simulink model "single_PID_Inverted_pendulum_Swingup"  (R2023b)
settings: Solver=FixedStepDiscrete  StartTime=0.0  StopTime=inf  FixedStep=0.005  RelTol=1e-3
undefined symbols (not defined in the file): Kd0, Ki0, Kp0
libraries: simulink x9, arduinolib x2, slpidlib x1
settings Model: ExtModeTrigDuration=2  Creator=ADMIN  LastModifiedBy=giabaomai
settings SolverCC: AutoInsertRateTranBlk=on
settings OptimizationCC: EnhancedBackFolding=on  PassReuseOutputArgsAs=Individual arguments  ZeroExternalMemoryAtStartup=off  ZeroInternalMemoryAtStartup=off  MaxStackSize=64  OptimizeBlockOrder=speed  DifferentSizesBufferReuse=on  EfficientTunableParamExpr=on
settings DebuggingCC: MultiTaskCondExecSysMsg=none  ParameterPrecisionLossMsg=none  ParameterTunabilityLossMsg=error
settings HardwareCC: ProdBitPerInt=16  ProdBitPerPointer=16  ProdBitPerSizeT=16  ProdBitPerPtrDiffT=16  ProdLargestAtomicFloat=None  ProdWordSize=8  ProdHWDeviceType=Atmel->AVR
settings SFSimCC: MATLABDynamicMemAlloc=off
settings RTWCC: Description=Embedded Coder  SystemTargetFile=ert.tlc  HardwareBoard=Arduino Mega 2560  TemplateMakefile=ert_default_tmf  Toolchain=Arduino AVR  BuildConfiguration=Faster Runs
settings CodeAppCC: ForceParamTrailComments=on  IgnoreCustomStorageClasses=off  OperatorAnnotations=on  SimulinkDataObjDesc=on  SFDataObjDesc=on  InsertBlockDesc=on
settings ERTTargetCC: SupportContinuousTime=on  SupportVariableSizeSignals=on  ExtModeTransport=3  ExtModeStaticAlloc=on  ExtModeAutomaticAllocSize=off  ExtModeStaticAllocSize=2048  ExtModeMexFile=ext_xcp  ExtModeIntrfLevel=Level2 - Open

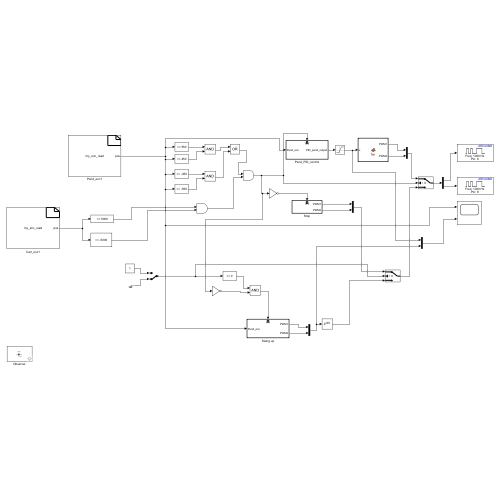
[thumbnail: Simulink's stored preview of the top-level diagram]
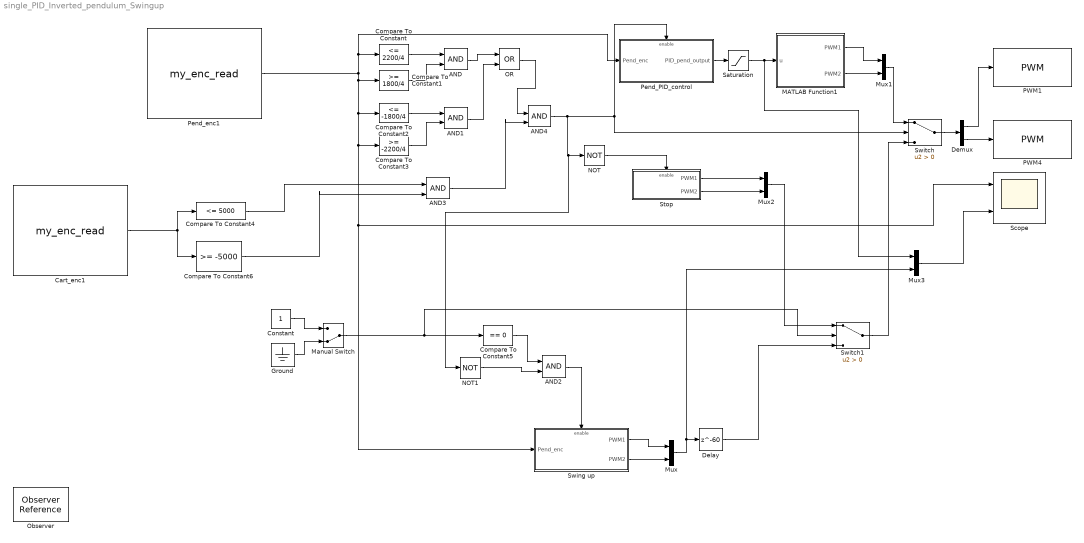
== system single_PID_Inverted_pendulum_Swingup ==
  AND : Logic  AllPortsSameDT=off  OutDataTypeStr=boolean
  AND1 : Logic  AllPortsSameDT=off  OutDataTypeStr=boolean
  AND2 : Logic  AllPortsSameDT=off  OutDataTypeStr=boolean
  AND3 : Logic  IconShape=distinctive  AllPortsSameDT=off  OutDataTypeStr=boolean
  AND4 : Logic  IconShape=distinctive  AllPortsSameDT=off  OutDataTypeStr=boolean
  Cart_enc1 : S-Function  FunctionName=my_enc_read  Parameters=uint8(3),uint8(2),uint8(0)  SFunctionModules=my_enc_read_wrapper.c  SFunctionDeploymentMode=off  EnableBusSupport=off  mask(S-Function Builder){}
      mask help: Simulink:masks:SFunctionBuilder_MD
      mask init:
      | val = [[.9  0.75 0.75 1 1 .9 .9 1]',[1 1 0.75 0.75 .9 .9 1 .9]'];try , sys = get_param(gcb,'SfunBuilderFcnName');if isempty(sys), sys = get_param(gcb,'FunctionName'); end,catch, sys = get_param(gcb,'FunctionName'); end
      settings: CopyFcn=set_param(gcbh,'LinkStatus','none')  OpenFcn=sfunctionwizard(gcbh)
      mask Display: plot(val(:,1),val(:,2)),disp(sys),port_label('output',1,'pos')
  Compare To Constant : simulink/Logic and Bit Operations/Compare To Constant  relop=<=  const=2200/4  OutDataTypeStr=boolean
  Compare To Constant1 : simulink/Logic and Bit Operations/Compare To Constant  relop=>=  const=1800/4  OutDataTypeStr=boolean
  Compare To Constant2 : simulink/Logic and Bit Operations/Compare To Constant  relop=<=  const=-1800/4  OutDataTypeStr=boolean
  Compare To Constant3 : simulink/Logic and Bit Operations/Compare To Constant  relop=>=  const=-2200/4  OutDataTypeStr=boolean
  Compare To Constant4 : simulink/Logic and Bit Operations/Compare To Constant  relop=<=  const=5000  OutDataTypeStr=boolean
  Compare To Constant5 : simulink/Logic and Bit Operations/Compare To Constant  relop===  const=0  OutDataTypeStr=boolean
  Compare To Constant6 : simulink/Logic and Bit Operations/Compare To Constant  relop=>=  const=-5000  OutDataTypeStr=boolean
  Constant : Constant
  Delay : Delay  DelayLength=60  SampleTime=0.005
  Demux : Demux  Outputs=2
  Ground : Ground
  MATLAB Function1 : MATLAB Function  TreatAsAtomicUnit=on
  Manual Switch : ManualSwitch  CurrentSetting=0
  Mux{,1..3} (4 alike) : Mux  Inputs=2
  NOT : Logic  Operator=NOT  IconShape=distinctive  AllPortsSameDT=off  OutDataTypeStr=boolean
  NOT1 : Logic  Operator=NOT  IconShape=distinctive  AllPortsSameDT=off  OutDataTypeStr=boolean
  OR : Logic  Operator=OR  AllPortsSameDT=off  OutDataTypeStr=boolean
  Observer : ObserverReference  ObserverModelName=single_PID_Inverted_pendulum_Swingup_Observer1
  PWM1 : arduinolib/PWM  pinNumber=6  frequencyType=Specify  desiredFrequency=1000  achievableFrequency=1000
  PWM4 : arduinolib/PWM  pinNumber=8  frequencyType=Specify  desiredFrequency=1000  achievableFrequency=1000
  Pend_PID_control : Subsystem  TreatAsAtomicUnit=on
  Pend_enc1 : S-Function  FunctionName=my_enc_read  Parameters=uint8(18),uint8(19),uint8(1)  SFunctionModules=my_enc_read_wrapper.c  SFunctionDeploymentMode=off  EnableBusSupport=off  mask(S-Function Builder){}
      mask help: Simulink:masks:SFunctionBuilder_MD
      mask init: same as single_PID_Inverted_pendulum_Swingup/Cart_enc1
      settings: CopyFcn=set_param(gcbh,'LinkStatus','none')  OpenFcn=sfunctionwizard(gcbh)
      mask Display:
      | plot(val(:,1),val(:,2))
      | disp(sys)
      | port_label('output',1,'pos')
  Saturation : Saturate  UpperLimit=255  LowerLimit=-255
  Scope : Scope  NumInputPorts=2
  Stop : Subsystem  TreatAsAtomicUnit=on
  Swing up : Subsystem  TreatAsAtomicUnit=on
  Switch : Switch  Criteria=u2 > Threshold  SaturateOnIntegerOverflow=off  InputSameDT=off
  Switch1 : Switch  Criteria=u2 > Threshold  SaturateOnIntegerOverflow=off  InputSameDT=off
  wires:
  MATLAB Function1/1(PWM1) -> Mux1/1
  Saturation/1 -> Mux3/1, MATLAB Function1/1(u)
  MATLAB Function1/2(PWM2) -> Mux1/2
  Pend_PID_control/1(PID_pend_output) -> Saturation/1
  Pend_enc1/1 -> Pend_PID_control/1(Pend_enc), Compare To Constant/1, Swing up/1(Pend_enc), Scope/1, Compare To Constant3/1, Compare To Constant2/1, Compare To Constant1/1
  Compare To Constant/1 -> AND/1
  Compare To Constant1/1 -> AND/2
  Compare To Constant2/1 -> AND1/1
  Compare To Constant3/1 -> AND1/2
  AND/1 -> OR/1
  AND1/1 -> OR/2
  NOT/1 -> Stop/Enable
  Stop/1(PWM1) -> Mux2/1
  Stop/2(PWM2) -> Mux2/2
  Mux1/1 -> Switch/1
  Switch/1 -> Demux/1
  Demux/1 -> PWM1/1
  Demux/2 -> PWM4/1
  Compare To Constant5/1 -> AND2/1
  NOT1/1 -> AND2/2
  Manual Switch/1 -> Switch1/2, Compare To Constant5/1
  AND2/1 -> Swing up/Enable
  Ground/1 -> Manual Switch/2
  Constant/1 -> Manual Switch/1
  Mux/1 -> Mux3/2, Delay/1
  Swing up/1(PWM1) -> Mux/1
  Swing up/2(PWM2) -> Mux/2
  Delay/1 -> Switch1/3
  Mux2/1 -> Switch1/1
  Switch1/1 -> Switch/3
  Mux3/1 -> Scope/2
  Cart_enc1/1 -> Compare To Constant4/1, Compare To Constant6/1
  Compare To Constant4/1 -> AND3/1
  Compare To Constant6/1 -> AND3/2
  OR/1 -> AND4/1
  AND3/1 -> AND4/2
  AND4/1 -> NOT1/1, NOT/1, Pend_PID_control/Enable, Switch/2

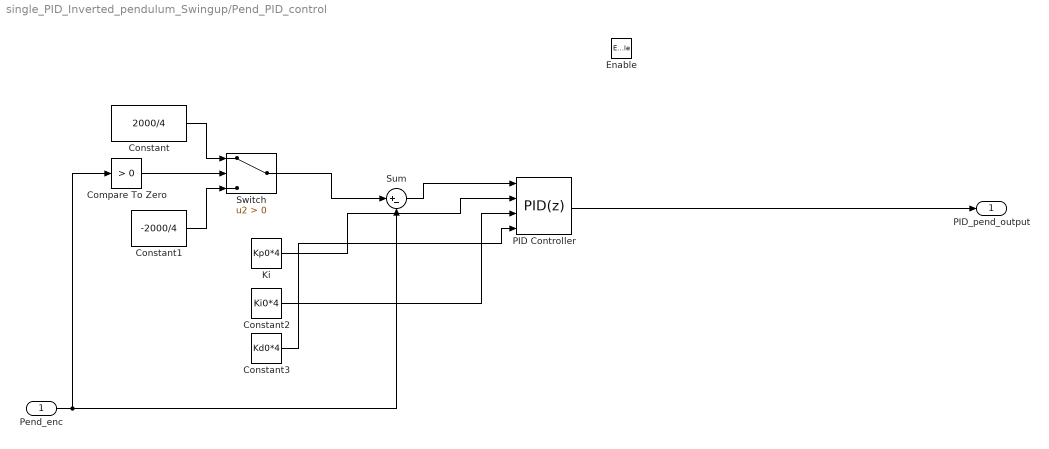
== system single_PID_Inverted_pendulum_Swingup/Pend_PID_control ==
  Pend_enc : Inport
  Enable : EnablePort
  Compare To Zero : simulink/Logic and Bit Operations/Compare To Zero  relop=>  OutDataTypeStr=boolean
  Constant : Constant  Value=2000/4
  Constant1 : Constant  Value=-2000/4
  Constant2 : Constant  Value=Ki0*4
  Constant3 : Constant  Value=Kd0*4
  Ki : Constant  Value=Kp0*4
  PID Controller : slpidlib/PID Controller  Controller=PID  Form=Parallel  TimeDomain=Discrete-time  UseExternalTs=off  SampleTime=0.005  IntegratorMethod=Backward Euler  FilterMethod=Forward Euler  ControllerParametersSource=external  P=0.35  I=0.12  UseKiTs=off  D=0.1  N=100  UseFilter=off  TunerSelectOption=Transfer Function Based (PID Tuner App)  ZeroCross=off  InitialConditionSource=internal  InitialConditionForIntegrator=0  InitialConditionForFilter=0  DifferentiatorICPrevScaledInput=0  ExternalReset=none  TrackingMode=off  Kt=1  LimitOutput=off  SatLimitsSource=internal  UpperSaturationLimit=255  LowerSaturationLimit=-255  LinearizeAsGain=off  AntiWindupMode=back-calculation  Kb=0.1  LimitIntegrator=off  UpperIntegratorSaturationLimit=inf  LowerIntegratorSaturationLimit=-inf  PGainOutDataTypeStr=Inherit: Match scaling  PProdOutDataTypeStr=Inherit: Match scaling  POutMin=[]  POutMax=[]  IOutMin=[]  IOutMax=[]  DOutMin=[]  DOutMax=[]  NOutMin=[]  NOutMax=[]  SumOutMin=[]  SumOutMax=[]  SaturationOutMin=[]  SaturationOutMax=[]  PParamMin=[]  PParamMax=[]  IParamMin=[]  IParamMax=[]  DParamMin=[]  DParamMax=[]  NParamMin=[]  NParamMax=[]  KbParamMin=[]  KbParamMax=[]  KtParamMin=[]  KtParamMax=[]  KbOutMin=[]  KbOutMax=[]  KtOutMin=[]  KtOutMax=[]  IntegratorOutMin=[]  IntegratorOutMax=[]  FilterOutMin=[]  FilterOutMax=[]  SumI1OutMin=[]  SumI1OutMax=[]  SumI2OutMin=[]  SumI2OutMax=[]  SumI3OutMin=[]  SumI3OutMax=[]  SumI4OutMin=[]  SumI4OutMax=[]  SumDOutMin=[]  SumDOutMax=[]  DifferentiatorOutMin=[]  DifferentiatorOutMax=[]  FilterDiffOutCoefMin=[]  FilterDiffOutCoefMax=[]  ReciprocalOutMin=[]  ReciprocalOutMax=[]  SumDenOutMin=[]  SumDenOutMax=[]  SumNumOutMin=[]  SumNumOutMax=[]  DivideOutMin=[]  DivideOutMax=[]  UdiffTsProdOutMin=[]  UdiffTsProdOutMax=[]  NTsProdOutMin=[]  NTsProdOutMax=[]  UintegralTsProdOutMin=[]  UintegralTsProdOutMax=[]  UngainTsProdOutMin=[]  UngainTsProdOutMax=[]  ClampingZeroOutDataTypeStr=Inherit: Inherit via back propagation  ClampingZeroOutMin=[]  ClampingZeroOutMax=[]  FilterDenConstantOutDataTypeStr=Inherit: Inherit via back propagation  FilterDenConstantOutMin=[]  FilterDenConstantOutMax=[]  PCopyOutDataTypeStr=Inherit: Inherit via back propagation  PCopyOutMin=[]  PCopyOutMax=[]  NCopyOutDataTypeStr=Inherit: Inherit via back propagation  NCopyOutMin=[]  NCopyOutMax=[]  IntegratorContinuousStateAttributes=''  IntegratorStateMustResolveToSignalObject=off  IntegratorRTWStateStorageClass=Auto  FilterContinuousStateAttributes=''  FilterStateMustResolveToSignalObject=off  FilterRTWStateStorageClass=Auto  ParallelPVariant=ExternalParameters  IdealPVariant=Disabled  IVariant=ExternalParameters  DVariant=ExternalParameters  IntegratorVariant=Discrete  SatVariant=Disabled  AWVariant=Passthrough  PCopyVariant=Disabled  TRVariant=Disabled  FdbkBlocksVariant=Forward  IdealPFdbkVariant=Disabled  SatFdbkVariant=Disabled  DerivativeFilterVariant=Differentiator  NVariant=Passthrough  NCopyVariant=Disabled_SignalSpec  FilterICVariant=InternalICsDifferentiator  IntegratorICVariant=InternalICs  ExternalResetVariant=Disabled  TRSumVariant=Passthrough  SumFdbkVariant=Disabled  SumVariant=Sum_PID  TsampFilterVariant=InternalTs  TsampNgainVariant=Passthrough  TsampIntegralVariant=Disabled_SignalSpec  ExternalSaturationOutDataTypeStr=Inherit: Same as second input
  Sum : Sum  Inputs=|+-
  Switch : Switch  Criteria=u2 > Threshold  SaturateOnIntegerOverflow=off  InputSameDT=off
  PID_pend_output : Outport
  wires:
  Ki/1 -> PID Controller/2
  Constant3/1 -> PID Controller/4
  Constant2/1 -> PID Controller/3
  Sum/1 -> PID Controller/1
  Pend_enc/1 -> Compare To Zero/1, Sum/2
  PID Controller/1 -> PID_pend_output/1
  Compare To Zero/1 -> Switch/2
  Constant/1 -> Switch/1
  Constant1/1 -> Switch/3
  Switch/1 -> Sum/1

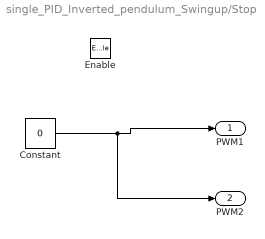
== system single_PID_Inverted_pendulum_Swingup/Stop ==
  Enable : EnablePort
  Constant : Constant  Value=0
  PWM1 : Outport
  PWM2 : Outport  Port=2
  wires:
  Constant/1 -> PWM2/1, PWM1/1

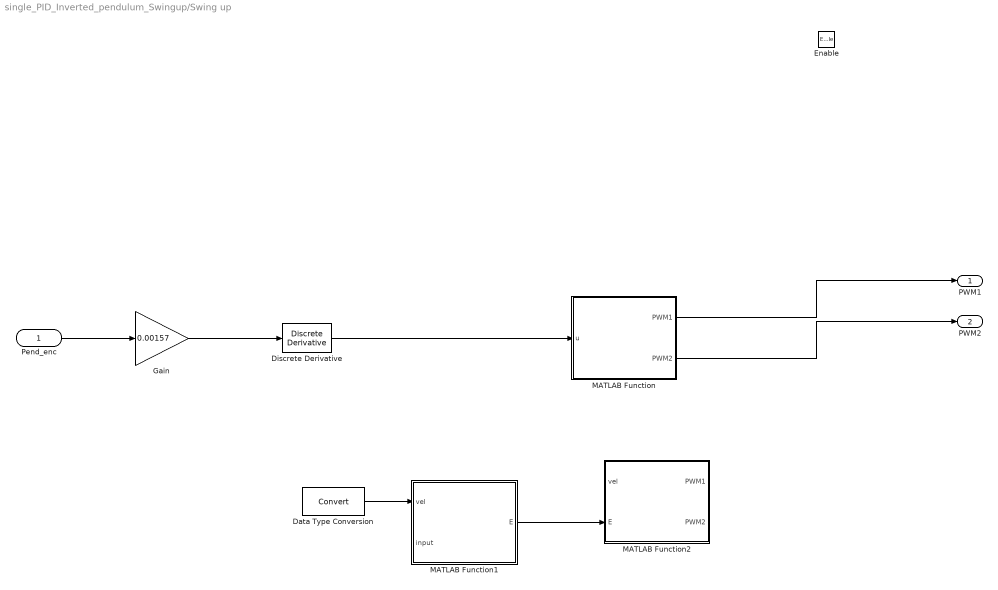
== system single_PID_Inverted_pendulum_Swingup/Swing up ==
  Pend_enc : Inport
  Enable : EnablePort
  Data Type Conversion : DataTypeConversion  SaturateOnIntegerOverflow=off  RndMeth=Floor
  Discrete Derivative : simulink/Discrete/Discrete Derivative  gainval=1.0  ICPrevScaledInput=0.0  InputProcessing=Columns as channels (frame based)  OutMin=[]  OutMax=[]  OutDataType=fixdt(1, 16)  OutScaling=2^-10  DoSatur=off
  Gain : Gain  Gain=0.00157
  MATLAB Function : MATLAB Function  TreatAsAtomicUnit=on
  MATLAB Function1 : MATLAB Function  TreatAsAtomicUnit=on
  MATLAB Function2 : MATLAB Function  TreatAsAtomicUnit=on
  PWM1 : Outport
  PWM2 : Outport  Port=2
  wires:
  Pend_enc/1 -> Gain/1
  Gain/1 -> Discrete Derivative/1
  MATLAB Function1/1(E) -> MATLAB Function2/2(E)
  Discrete Derivative/1 -> MATLAB Function/1(u)
  MATLAB Function/1(PWM1) -> PWM1/1
  MATLAB Function/2(PWM2) -> PWM2/1
  Data Type Conversion/1 -> MATLAB Function1/1(vel)

== matlab function single_PID_Inverted_pendulum_Swingup/Swing up/MATLAB Function ==
  data: u input; PWM1 output; PWM2 output
function [PWM1, PWM2] = fcn(u)
if (u>0)
  PWM1 = 40;
  PWM2 = 0;
else (u<=0);
  PWM1 = 0;
  PWM2 = 40;
end

== matlab function single_PID_Inverted_pendulum_Swingup/MATLAB Function1 ==
  data: u input; PWM1 output; PWM2 output
function [PWM1, PWM2] = fcn(u)
if u<0
  PWM1 = abs(u);
  PWM2 = 0;
elseif u>0
  PWM1 =0;
  PWM2 =abs(u);
else u=0;
  PWM1 = 0;
  PWM2 = 0;
end

== matlab function single_PID_Inverted_pendulum_Swingup/Swing up/MATLAB Function1 ==
  data: vel input; E output; input input
function E = fcn(vel,input)
m=0.1;
l=0.2;
g=9.81;
E=(1/2)*m*(l^2)*((vel)^2)+m*g*l*(1-cos(input));

== matlab function single_PID_Inverted_pendulum_Swingup/Swing up/MATLAB Function2 ==
  data: vel input; PWM1 output; PWM2 output; E input
function [PWM1, PWM2] = fcn(vel,E)

if (vel<0 && E<4.2) || (vel>=0 && E>=4.2)
  PWM1 = 30;
  PWM2 = 0;
else (vel>=0 && E<4.2) || (vel<0 && E>=4.2);
  PWM1 = 0;
  PWM2 = 30;
end
